simulink model "process_model_2"  (R2023b)
settings: Solver=FixedStepDiscrete  StartTime=0.0  StopTime=10.0  RelTol=1e-3
values from neighbouring files (symbols this model uses):
  samp_t = 1    [ca2_params.m]    (also in iterate_gains.m)
undefined symbols (not defined in the file or in its folder): a_2, b_2, d_2
settings Model: Creator=john  LastModifiedBy=john

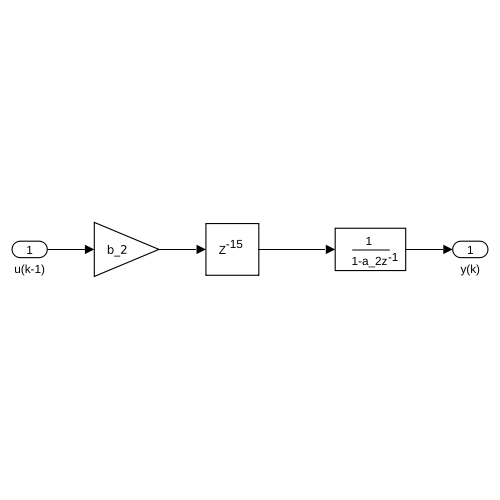
[thumbnail: Simulink's stored preview of the top-level diagram]
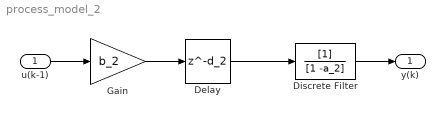
== system process_model_2 ==
  u(k-1) : Inport
  Delay : Delay  DelayLength=d_2  SampleTime=samp_t
  Discrete Filter : DiscreteFilter  Denominator=[1 -a_2]
  Gain : Gain  Gain=b_2
  y(k) : Outport
  wires:
  Delay/1 -> Discrete Filter/1
  Gain/1 -> Delay/1
  u(k-1)/1 -> Gain/1
  Discrete Filter/1 -> y(k)/1
